simulink model "m_frig"  (Simulink 10.0)
settings: Solver=ode15s  StartTime=0.0  StopTime=5000  FixedStep=.1  RelTol=1e-5  EnableMultiTasking=on
settings Model: Creator=prof. G. Celentano  LastModifiedBy=AR  ExtModeTrigMode=oneshot  ExtModeArmWhenConnect=off
settings DataIOCC: SignalLoggingSaveFormat=ModelDataLogs  SignalLoggingName=sigsOut
settings OptimizationCC: BooleanDataType=off  ExpressionDepthLimit=2147483647
settings DebuggingCC: SaveWithParameterizedLinksMsg=none  SignalResolutionControl=TryResolveAllWithWarning  MultiTaskDSMMsg=warning  MultiTaskCondExecSysMsg=none  FcnCallInpInsideContextMsg=warning  StateNameClashWarn=warning
settings HardwareCC: TargetUnknown=on

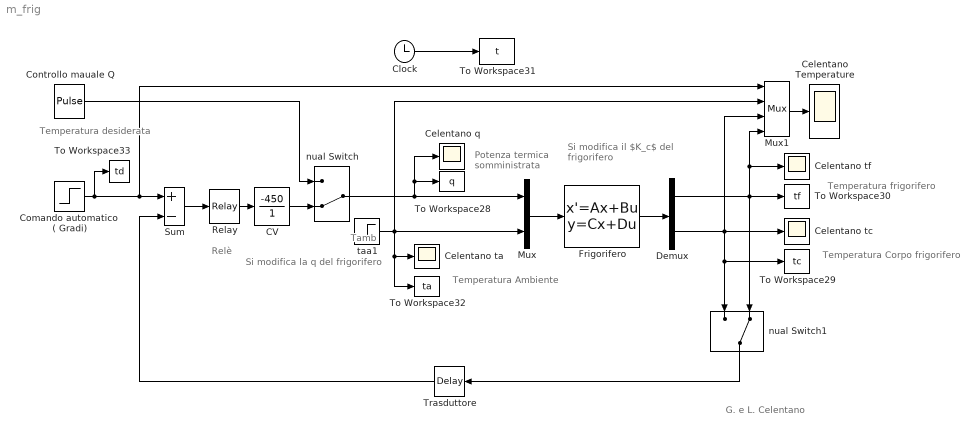
== system m_frig ==
  note: Relè
  note: Potenza
      | termica
      | somministrata
  note: Si modifica la q
      | del frigorifero
  note: Si modifica il $K_c$
      | del frigorifero
  note: Tamb
  note: G. e L. Celentano
  note: Temperatura
      | Ambiente
  note: Temperatura
      | Corpo frigorifero
  note: Temperatura
      | desiderata
  note: Temperatura
      | frigorifero
  " Trasduttore" : TransportDelay
  CV : TransferFcn  Numerator=-450  Denominator=1
  Celentano Temperature : Scope
  Celentano q : Scope
  Celentano ta : Scope
  Celentano tc : Scope
  Celentano tf : Scope
  Clock : Clock
  Comando automatico  ( Gradi) : Step  Time=2500  After=5  SampleTime=0
  Controllo mauale Q : DiscretePulseGenerator  PulseType=Time based  Amplitude=-1000  Period=2000  PulseWidth=75
  Demux : Demux  Outputs=2
  Frigorifero : StateSpace  A="[-(25+5)/5e3  5/5e3; 5/1e3  -5/1e3]"  B="[1/5e3  25/5e3; 0  0]"  C=eye(2)  D=zeros(2, 2)  InitialCondition="[30  30]"
  Mux : Mux  Inputs=2
  Mux1 : Mux
  Relay : Relay  OnSwitchValue=.5  OffSwitchValue=-.5  OnOutputValue=0  OffOutputValue=1
  Sum : Sum  Inputs=+-  SaturateOnIntegerOverflow=on  InputSameDT=on  OutDataTypeStr=Inherit: Same as first input
  To Workspace28 : ToWorkspace  VariableName=q  SampleTime=-1
  To Workspace29 : ToWorkspace  VariableName=tc  SampleTime=-1
  To Workspace30 : ToWorkspace  VariableName=tf  SampleTime=-1
  To Workspace31 : ToWorkspace  VariableName=t  SampleTime=-1
  To Workspace32 : ToWorkspace  VariableName=ta  SampleTime=-1
  To Workspace33 : ToWorkspace  VariableName=td  SampleTime=-1
  nual Switch : ManualSwitch  CurrentSetting=0
  nual Switch1 : ManualSwitch  CurrentSetting=0
  taa1 : Step  Time=2500  Before=30  After=20  SampleTime=0
  wires:
  taa1/1 -> Celentano ta/1, To Workspace32/1, Mux/2, Mux1/2
  nual Switch/1 -> Celentano q/1, To Workspace28/1, Mux/1
  CV/1 -> nual Switch/2
  Mux1/1 -> Celentano Temperature/1
  Demux/1 -> To Workspace30/1, nual Switch1/2, Celentano tf/1, Mux1/4
  Demux/2 -> Celentano tc/1, Mux1/3, nual Switch1/1, To Workspace29/1
  Mux/1 -> Frigorifero/1
  Frigorifero/1 -> Demux/1
  nual Switch1/1 -> " Trasduttore"/1
  Clock/1 -> To Workspace31/1
  Sum/1 -> Relay/1
  Relay/1 -> CV/1
  Comando automatico  ( Gradi)/1 -> Sum/1, Mux1/1, To Workspace33/1
  " Trasduttore"/1 -> Sum/2
  Controllo mauale Q/1 -> nual Switch/1
